simulink model "MotorCC_chopperPWM"  (R2024b)
settings: Solver=ode45  StartTime=0.0  StopTime=0.5  RelTol=1e-3  EnableMultiTasking=on
InitFcn:
  | Tsim = 1;
  | Ra = 0.71218;
  | La = 4.2915e-04;
  | J = 0.00015263;
  | B = 0.00045348;
  | K = 0.072987;
  | TC = 0;
  | Va = 12.4; % Barramento CC %
libraries: simulink x1, spsDCMachineLib x1, spsDCVoltageSourceLib x1, spsDiodeLib x1, spsIGBTLib x1, spsMeanLib x1, spsSawtoothGeneratorLib x1, cstblocks x1, sps_lib x1, spsVoltageMeasurementLib x1
settings Model: Creator=Lucas Jonys  LastModifiedBy=leocs
settings SolverCC: AlgebraicLoopSolver=TrustRegion
settings DataIOCC: ReturnWorkspaceOutputs=off
settings OptimizationCC: LifeSpan=inf
settings DebuggingCC: UnconnectedInputMsg=warning  UnconnectedOutputMsg=warning  UnconnectedLineMsg=warning  SFUnexpectedBacktrackingDiag=warning  SFNoUnconditionalDefaultTransitionDiag=warning  ArithmeticOperatorsInVariantConditions=warning
settings ModelReferenceCC: EnableRefExpFcnMdlSchedulingChecks=on
settings SFSimCC: SimUseLocalCustomCode=off  CustomCodeUndefinedFunction=UseInterfaceOnly
settings RTWCC: RTWUseLocalCustomCode=off  GPUComputeCapability=3.5
settings CodeAppCC: StateflowObjectComments=on
settings GRTTargetCC: TargetLangStandard=C89/C90 (ANSI)
settings ConfigComp: CovMetricSettings=dw  CovSaveCumulativeToWorkspaceVar=on  CovSaveSingleToWorkspaceVar=on  CovExternalEMLEnable=off
settings SimscapeCC: SimscapeNormalizeSystem=off

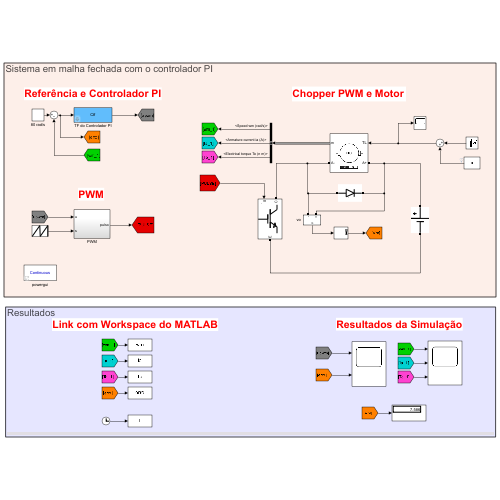
[thumbnail: Simulink's stored preview of the top-level diagram]
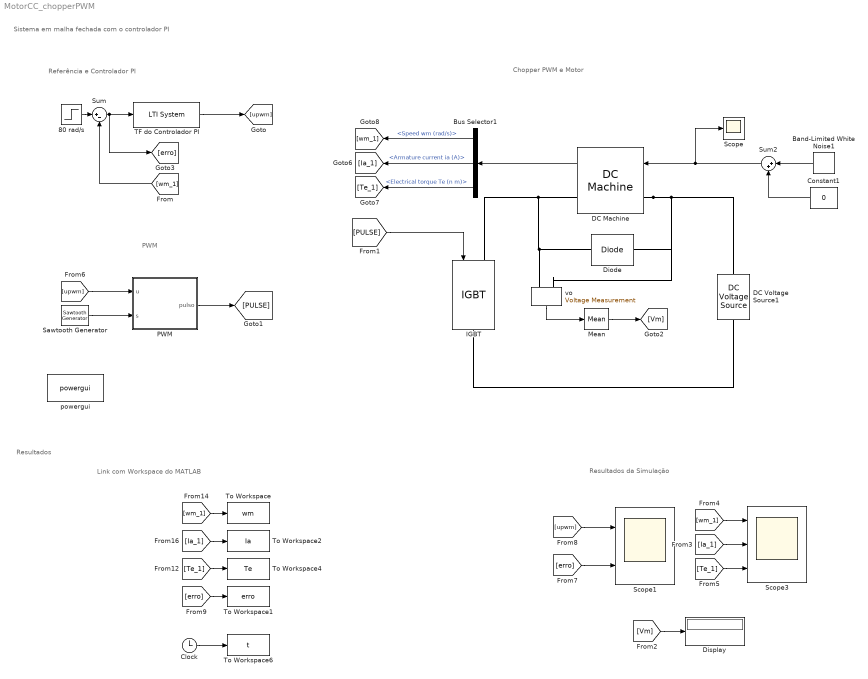
== system MotorCC_chopperPWM ==
  note: Resultados
  note: Sistema em malha fechada com o controlador PI
  note: Resultados da Simulação
  note: Chopper PWM e Motor
  note: Link com Workspace do MATLAB
  note: PWM
  note: Referência e Controlador PI
  80 rad/s : Step  Time=0  After=80  SampleTime=0
  Band-Limited White Noise1 : simulink/Sources/Band-Limited White Noise  Cov=[0.0000000]  Ts=0.0000005  seed=[23341]
  Bus Selector1 : BusSelector  OutputSignals=Speed wm (rad/s),Armature current ia (A),Electrical torque Te (n m)
  Clock : Clock
  Constant1 : Constant  Value=0
  DC Machine : spsDCMachineLib/DC Machine  PresetModel=No  MechanicalLoad=Torque TL  FieldType=Permanent magnet  ShowDetailedParameters=on  MeasurementBus=off  RLa=[2.8731 0.0047]  RLf="[ 240  120]"  Laf=1.8  MachineConstant=Torque constant (N.m/A)  Ke=1.8  Kt=0.0870  J=5.5388e-05  Bm=2.3689e-04  Tf=0  w0=0  Ifinit=1  TsPowergui=0  TsBlock=-1
  DC Voltage Source1 : spsDCVoltageSourceLib/DC Voltage Source  Amplitude=Va  Measurements=None
  Diode : spsDiodeLib/Diode  Ron=0.15  Lon=0  Vf=0.7  IC=0  UseSnubber=off  Rs=inf  Cs=inf  Measurements=off
  Display : Display
  IGBT : spsIGBTLib/IGBT  Ron=0.01  Lon=0  Vf=0  Tf=1e-6  Tt=2e-6  IC=0  Rs=inf  Cs=inf  Measurements=off
  Mean : spsMeanLib/Mean  Freq=4000  Vinit=0  Ts=0
  PWM : Subsystem
  Sawtooth Generator : spsSawtoothGeneratorLib/Sawtooth Generator  Freq=4000  Phase=0  Ts=0
  Scope : Scope
  Scope1 : Scope  NumInputPorts=2
  Scope3 : Scope  NumInputPorts=3
  Sum : Sum  Inputs=|+-
  Sum2 : Sum  Inputs=|++
  TF do Controlador PI : cstblocks/LTI System  sys=Ctf  IC=[]  PadeOrder=0
  To Workspace : ToWorkspace  VariableName=wm  SampleTime=-1
  To Workspace1 : ToWorkspace  VariableName=erro  SampleTime=-1
  To Workspace2 : ToWorkspace  VariableName=Ia  SampleTime=-1
  To Workspace4 : ToWorkspace  VariableName=Te  SampleTime=-1
  To Workspace6 : ToWorkspace  VariableName=t  SampleTime=-1
  powergui : sps_lib/powergui  Priority=1  SimulationMode=Continuous  SampleTime=50e-6  frequency=60  Iterations=50  frequencyindice=0  Pbase=100e6  ErrMax=1e-4  UnitsV=kV  UnitsW=MW  buscounter=0  FunctionMessages=off  echomessages=off  EnableUseOfTLC=off  CurrentSourceSwitches=off  DisableSnubberDevices=off  DisableRonSwitches=off  DisableVfSwitches=off  DisplayEquations=off  AutomaticDiscreteSolvers=off  SolverType=Tustin/Backward Euler (TBE)  Interpol=off  ExternalGateDelay=off  methode=off  Ts=100  x0status=blocks  SPID=on  SwTol=0  HookPort=off  NonlinearTolerance=1e-4  nMaxIteration=100  ContinueOnMaxIteration=off  RestoreLinks=warning  ResistiveCurrentMeasurement=off  Frange=[0:2:500]  Ylog=off  Xlog=on  ShowGrid=off  save=off  variable=ZData  structure=0  ZoomFFT=off  StartTime=0.0  cycles=1  DisplayStyle=1  fundamental=60  FreqAxis=off  MaxFrequency=1000  frequencyindicesteady=1  RmsSteady=1  display=off
  vo : spsVoltageMeasurementLib/Voltage Measurement  PhasorSimulation=off  OutputType=Complex  PSBequivalent=0
  wires:
  [wm_1] -> Scope3/1
  [Te_1] -> Scope3/3
  [Ia_1] -> Scope3/2
  [Te_1] -> To Workspace4/1
  [wm_1] -> To Workspace/1
  [Ia_1] -> To Workspace2/1
  Clock/1 -> To Workspace6/1
  [Vm] -> Display/1
  vo/1 -> Mean/1
  Mean/1 -> [Vm]
  DC Machine/1 -> Bus Selector1/1
  Bus Selector1/1 -> [wm_1]  "<Speed wm (rad/s)>"
  Bus Selector1/2 -> [Ia_1]  "<Armature current ia (A)>"
  Bus Selector1/3 -> [Te_1]  "<Electrical torque Te (n m)>"
  [upwm] -> PWM/1(u)
  PWM/1(pulso) -> [PULSE]
  [PULSE] -> IGBT/1
  Sawtooth Generator/1 -> PWM/2(s)
  Constant1/1 -> Sum2/2
  Sum2/1 -> Scope/1, DC Machine/1
  Band-Limited White Noise1/1 -> Sum2/1
  80 rad/s/1 -> Sum/1
  Sum/1 -> [erro], TF do Controlador PI/1
  [wm_1] -> Sum/2
  [upwm] -> Scope1/1
  [erro] -> Scope1/2
  [erro] -> To Workspace1/1
  TF do Controlador PI/1 -> [upwm]
  connections:
  DC Machine/LConn1 -- Diode/RConn1 -- vo/LConn1 -- DC Voltage Source1/RConn1
  Diode/LConn1 -- vo/LConn2 -- DC Machine/RConn1 -- IGBT/LConn1
  IGBT/RConn1 -- DC Voltage Source1/LConn1

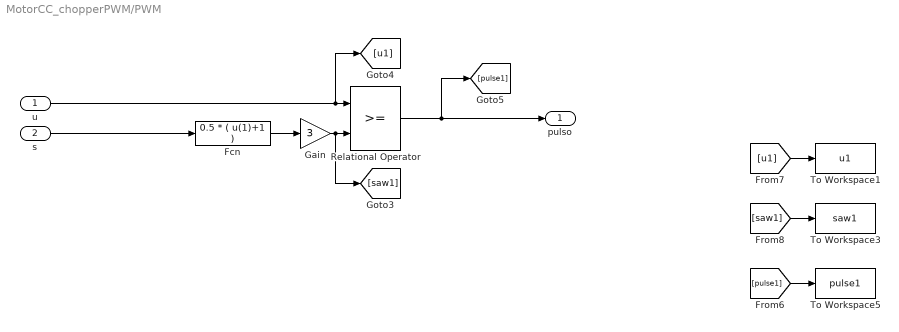
== system MotorCC_chopperPWM/PWM ==
  u : Inport
  s : Inport  Port=2
  Fcn : Fcn  Expr=0.5 * ( u(1)+1 )
  Gain : Gain  Gain=3
  Relational Operator : RelationalOperator  OutDataTypeStr=boolean  InputSameDT=off
  To Workspace1 : ToWorkspace  VariableName=u1  SampleTime=-1
  To Workspace3 : ToWorkspace  VariableName=saw1  SampleTime=-1
  To Workspace5 : ToWorkspace  VariableName=pulse1  SampleTime=-1
  pulso : Outport
  wires:
  Fcn/1 -> Gain/1
  s/1 -> Fcn/1
  Relational Operator/1 -> [pulse1], pulso/1
  u/1 -> [u1], Relational Operator/1
  Gain/1 -> [saw1], Relational Operator/2
  [u1] -> To Workspace1/1
  [pulse1] -> To Workspace5/1
  [saw1] -> To Workspace3/1
